simulink model "TempomatV1_2016"  (R2018b)
settings: Solver=FixedStepAuto  StartTime=0.0  StopTime=100.0  FixedStep=0.001  RelTol=1e-3
settings Model: Creator=marci  LastModifiedBy=marci
settings OptimizationCC: LifeSpan=inf
settings CodeAppCC: StateflowObjectComments=on

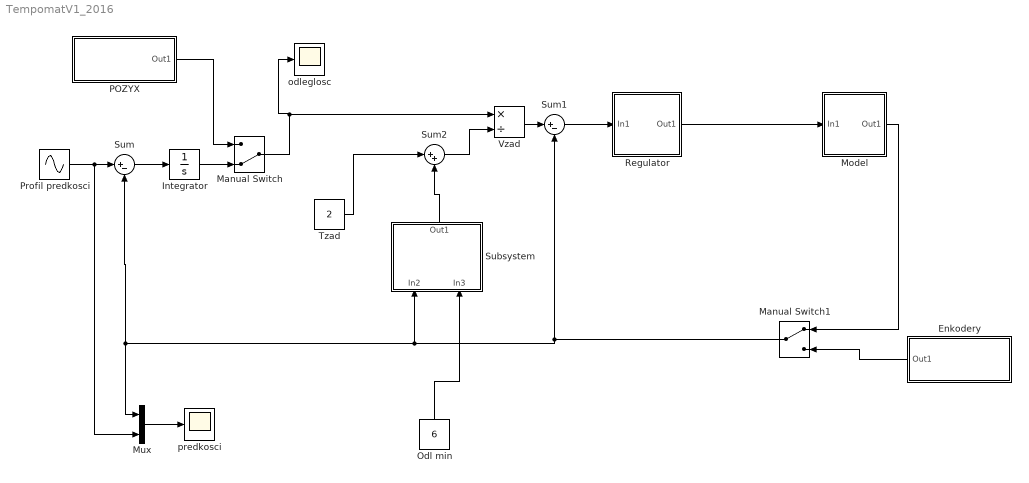
== system TempomatV1_2016 ==
  Enkodery : Subsystem
  Integrator : Integrator  InitialCondition=3
  Manual Switch : ManualSwitch  CurrentSetting=0
  Manual Switch1 : ManualSwitch
  Model : Subsystem
  Mux : Mux  Inputs=2
  Odl min : Constant  Value=6
  POZYX : Subsystem
  Profil predkosci : Sin  Amplitude=0.5  Bias=6  Frequency=0.5  SampleTime=0
  Regulator : Subsystem
  Subsystem : Subsystem
  Sum : Sum  Inputs=|+-
  Sum1 : Sum  Inputs=|+-
  Sum2 : Sum  Inputs=|++
  Tzad : Constant  Value=2
  Vzad : Product  Inputs=*/
  "odleglosc " : Scope
  predkosci : Scope
  wires:
  Sum/1 -> Integrator/1
  Mux/1 -> predkosci/1
  Sum1/1 -> Regulator/1(In1)
  Model/1(Out1) -> Manual Switch1/1
  Manual Switch1/1 -> Sum/2, Mux/1, Subsystem/1(In2), Sum1/2
  Integrator/1 -> Manual Switch/2
  POZYX/1(Out1) -> Manual Switch/1
  Profil predkosci/1 -> Mux/2, Sum/1
  Manual Switch/1 -> Vzad/1, "odleglosc "/1
  Enkodery/1(Out1) -> Manual Switch1/2
  Tzad/1 -> Sum2/1
  Sum2/1 -> Vzad/2
  Vzad/1 -> Sum1/1
  Regulator/1(Out1) -> Model/1(In1)
  Odl min/1 -> Subsystem/2(In3)
  Subsystem/1(Out1) -> Sum2/2

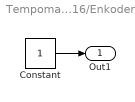
== system TempomatV1_2016/Enkodery ==
  Constant : Constant
  Out1 : Outport
  wires:
  Constant/1 -> Out1/1

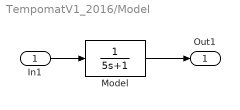
== system TempomatV1_2016/Model ==
  In1 : Inport
  Model : TransferFcn  Denominator=[5 1]
  Out1 : Outport
  wires:
  In1/1 -> Model/1
  Model/1 -> Out1/1

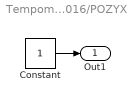
== system TempomatV1_2016/POZYX ==
  Constant : Constant
  Out1 : Outport
  wires:
  Constant/1 -> Out1/1

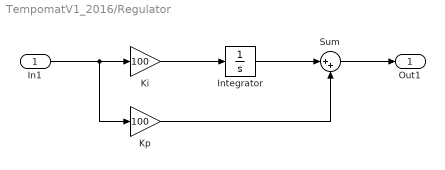
== system TempomatV1_2016/Regulator ==
  In1 : Inport
  Integrator : Integrator
  Ki : Gain  Gain=100
  Kp : Gain  Gain=100
  Sum : Sum  Inputs=|++
  Out1 : Outport
  wires:
  Ki/1 -> Integrator/1
  In1/1 -> Kp/1, Ki/1
  Sum/1 -> Out1/1
  Kp/1 -> Sum/2
  Integrator/1 -> Sum/1

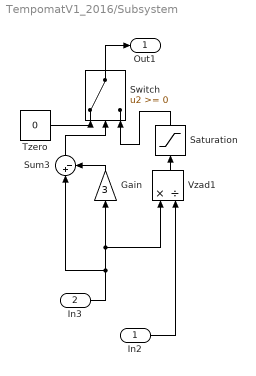
== system TempomatV1_2016/Subsystem ==
  In2 : Inport
  In3 : Inport  Port=2
  Gain : Gain  Gain=3
  Saturation : Saturate  UpperLimit=20  LowerLimit=0
  Sum3 : Sum  Inputs=|+-
  Switch : Switch
  Tzero : Constant  Value=0
  Vzad1 : Product  Inputs=*/
  Out1 : Outport
  wires:
  Sum3/1 -> Switch/2
  Vzad1/1 -> Saturation/1
  Gain/1 -> Sum3/2
  In3/1 -> Sum3/1, Gain/1, Vzad1/1
  In2/1 -> Vzad1/2
  Tzero/1 -> Switch/1
  Saturation/1 -> Switch/3
  Switch/1 -> Out1/1
